simulink model "MCU_FOC"  (R2022b)
settings: Solver=FixedStepDiscrete  StartTime=0.0  StopTime=10.0  FixedStep=0.0001  RelTol=1e-3
values from neighbouring files (symbols this model uses):
  C_FOC_DecoupleEn_u8 = 0.0    [MCU_FOC_Sldd.sldd]    (also in MCU_FOC_Sldd_objects.m = myPackage.Parameter)
  C_FOC_DecoupleUdCoeff_f32 = 0.0    [MCU_FOC_Sldd.sldd]    (also in MCU_FOC_Sldd_objects.m = myPackage.Parameter)
  C_FOC_DecoupleUeCoeff_f32 = 0.0    [MCU_FOC_Sldd.sldd]    (also in MCU_FOC_Sldd_objects.m = myPackage.Parameter)
  C_FOC_DecoupleUqCoeff_f32 = 0.0    [MCU_FOC_Sldd.sldd]    (also in MCU_FOC_Sldd_objects.m = myPackage.Parameter)
  C_FOC_DPWMEN_u8 = 0.0    [MCU_FOC_Sldd.sldd]    (also in MCU_FOC_Sldd_objects.m = myPackage.Parameter)
  C_FOC_IgnoreShunt_u8 = 0.0    [MCU_FOC_Sldd.sldd]    (also in MCU_FOC_Sldd_objects.m = myPackage.Parameter)
  C_FOC_ThetaOffsetCoeff_f32 = 0.0    [MCU_FOC_Sldd.sldd]    (also in MCU_FOC_Sldd_objects.m = myPackage.Parameter)
undefined symbols (not defined in the file or in its folder): ABC_SAMPLE, ANALOG, cAgeingMode, cParaRecogMode, cSingleBoardMode, cVvvfOpenMode, MAIN_CPU_FRE, ParamCfg_BaseSpeed_u16, ParamCfg_CommandSource_u16, ParamCfg_IdKi_u16, ParamCfg_IdKp_u16, ParamCfg_IdStep1_u16, ParamCfg_IdStep2_u16, ParamCfg_IqKi_u16, ParamCfg_IqKp_u16, ParamCfg_IqStep_u16, ParamCfg_MotorLsd_u16, ParamCfg_MotorNp_u16, ParamCfg_MotorUlsq_u16, ParamCfg_PwmFreqHigh_u16, ParamCfg_PwmFreqLow_u16, ParamCfg_Pwmprdchgen_u16, ParamCfg_RotateNp_u16, ParamCfg_RotorFlux_u16, ParamCfg_SampleMode_u16, TESTBED
libraries: simulink x40, YS_UserDefined_Library x17
(part 2 of 2)

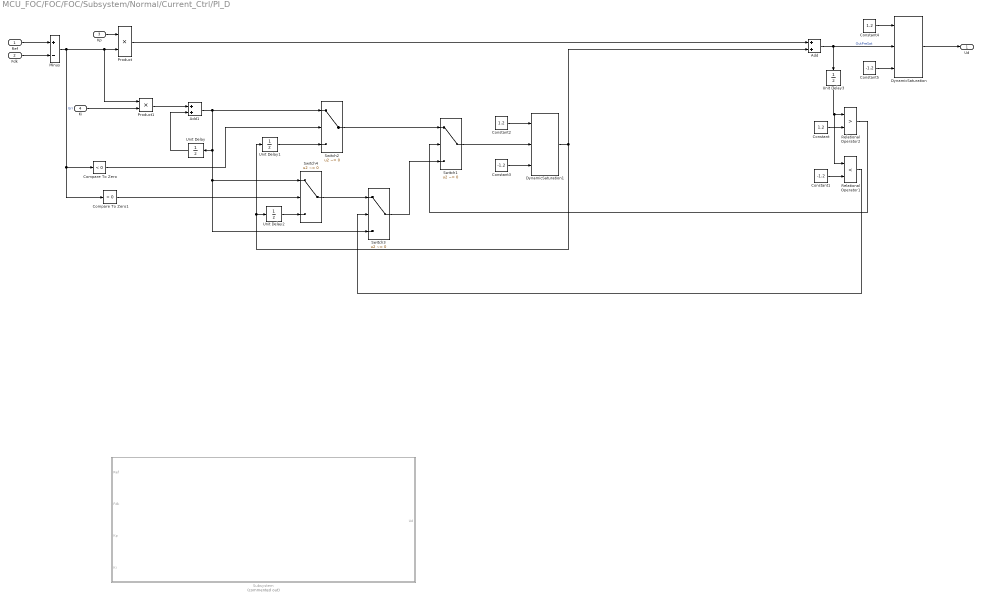
== system MCU_FOC/FOC/FOC/Subsystem/Normal/Current_Ctrl/PI_D ==
  Ref : Inport
  Fdk : Inport  Port=2
  Kp : Inport  Port=3
  Ki : Inport  Port=4
  Add : Sum
  Add1 : Sum
  Compare To Zero : simulink/Logic and Bit Operations/Compare To Zero  relop=<  OutDataTypeStr=boolean
  Compare To Zero1 : simulink/Logic and Bit Operations/Compare To Zero  relop=>  OutDataTypeStr=boolean
  Constant : Constant  Value=1.2  OutDataTypeStr=single
  Constant1 : Constant  Value=-1.2  OutDataTypeStr=single
  Constant2 : Constant  Value=1.2  OutDataTypeStr=single
  Constant3 : Constant  Value=-1.2  OutDataTypeStr=single
  Constant4 : Constant  Value=1.2  OutDataTypeStr=single
  Constant5 : Constant  Value=-1.2  OutDataTypeStr=single
  DynamicSaturation : YS_UserDefined_Library/Saturation/DynamicSaturation
      settings: SourceProductName=YS
  DynamicSaturation1 : YS_UserDefined_Library/Saturation/DynamicSaturation
      settings: SourceProductName=YS
  Minus : Sum  Inputs=+-
  Product : Product
  Product1 : Product
  Relational Operator1 : RelationalOperator  Operator=<  OutDataTypeStr=boolean  RndMeth=Simplest  InputSameDT=off
  Relational Operator2 : RelationalOperator  Operator=>  OutDataTypeStr=boolean  RndMeth=Simplest  InputSameDT=off
  Subsystem : Subsystem  Commented=on
  Switch{1..4} (4 alike) : Switch  Criteria=u2 ~= 0  SaturateOnIntegerOverflow=off  InputSameDT=off
  Unit Delay{,1..3} (4 alike) : UnitDelay  SampleTime=-1  HasFrameUpgradeWarning=on
  Ud : Outport
  wires:
  Constant2/1 -> DynamicSaturation1/1
  Constant/1 -> Relational Operator2/2
  Product/1 -> Add/1
  Ki/1 -> Product1/2
  Compare To Zero/1 -> Switch2/2
  DynamicSaturation1/1 -> Unit Delay1/1, Unit Delay2/1, Add/2
  Switch4/1 -> Switch3/1
  Unit Delay/1 -> Add1/2
  Switch2/1 -> Switch1/1
  Switch3/1 -> Switch1/3
  Compare To Zero1/1 -> Switch4/2
  Relational Operator1/1 -> Switch3/2
  Constant3/1 -> DynamicSaturation1/3
  Switch1/1 -> DynamicSaturation1/2
  Add1/1 -> Switch3/3, Switch4/1, Unit Delay/1, Switch2/1
  Unit Delay1/1 -> Switch2/3
  Add/1 -> DynamicSaturation/2, Unit Delay3/1  "OutPreSat"
  DynamicSaturation/1 -> Ud/1
  Product1/1 -> Add1/1
  Unit Delay2/1 -> Switch4/3
  Constant1/1 -> Relational Operator1/2
  Kp/1 -> Product/1
  Ref/1 -> Minus/1
  Minus/1 -> Product1/1, Product/2, Compare To Zero1/1, Compare To Zero/1  "Err"
  Fdk/1 -> Minus/2
  Constant4/1 -> DynamicSaturation/1
  Constant5/1 -> DynamicSaturation/3
  Relational Operator2/1 -> Switch1/2
  Unit Delay3/1 -> Relational Operator2/1, Relational Operator1/1

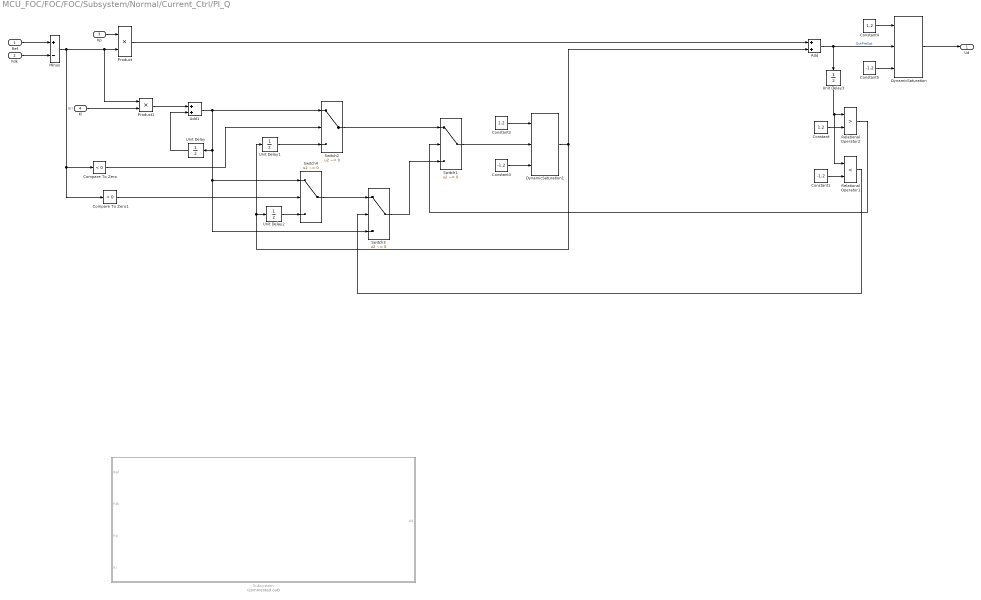
== system MCU_FOC/FOC/FOC/Subsystem/Normal/Current_Ctrl/PI_Q ==
  Ref : Inport
  Fdk : Inport  Port=2
  Kp : Inport  Port=3
  Ki : Inport  Port=4
  Add : Sum
  Add1 : Sum
  Compare To Zero : simulink/Logic and Bit Operations/Compare To Zero  relop=<  OutDataTypeStr=boolean
  Compare To Zero1 : simulink/Logic and Bit Operations/Compare To Zero  relop=>  OutDataTypeStr=boolean
  Constant : Constant  Value=1.2  OutDataTypeStr=single
  Constant1 : Constant  Value=-1.2  OutDataTypeStr=single
  Constant2 : Constant  Value=1.2  OutDataTypeStr=single
  Constant3 : Constant  Value=-1.2  OutDataTypeStr=single
  Constant4 : Constant  Value=1.2  OutDataTypeStr=single
  Constant5 : Constant  Value=-1.2  OutDataTypeStr=single
  DynamicSaturation : YS_UserDefined_Library/Saturation/DynamicSaturation
      settings: SourceProductName=YS
  DynamicSaturation1 : YS_UserDefined_Library/Saturation/DynamicSaturation
      settings: SourceProductName=YS
  Minus : Sum  Inputs=+-
  Product : Product
  Product1 : Product
  Relational Operator1 : RelationalOperator  Operator=<  OutDataTypeStr=boolean  RndMeth=Simplest  InputSameDT=off
  Relational Operator2 : RelationalOperator  Operator=>  OutDataTypeStr=boolean  RndMeth=Simplest  InputSameDT=off
  Subsystem : Subsystem  Commented=on
  Switch{1..4} (4 alike) : Switch  Criteria=u2 ~= 0  SaturateOnIntegerOverflow=off  InputSameDT=off
  Unit Delay{,1..3} (4 alike) : UnitDelay  SampleTime=-1  HasFrameUpgradeWarning=on
  Ud : Outport
  wires:
  Unit Delay3/1 -> Relational Operator1/1, Relational Operator2/1
  Relational Operator2/1 -> Switch1/2
  Constant5/1 -> DynamicSaturation/3
  Constant4/1 -> DynamicSaturation/1
  Fdk/1 -> Minus/2
  Minus/1 -> Compare To Zero/1, Compare To Zero1/1, Product/2, Product1/1  "Err"
  Ref/1 -> Minus/1
  Kp/1 -> Product/1
  Constant1/1 -> Relational Operator1/2
  Unit Delay2/1 -> Switch4/3
  Product1/1 -> Add1/1
  DynamicSaturation/1 -> Ud/1
  Add/1 -> Unit Delay3/1, DynamicSaturation/2  "OutPreSat"
  Unit Delay1/1 -> Switch2/3
  Add1/1 -> Switch2/1, Unit Delay/1, Switch4/1, Switch3/3
  Switch1/1 -> DynamicSaturation1/2
  Constant3/1 -> DynamicSaturation1/3
  Relational Operator1/1 -> Switch3/2
  Compare To Zero1/1 -> Switch4/2
  Switch3/1 -> Switch1/3
  Switch2/1 -> Switch1/1
  Unit Delay/1 -> Add1/2
  Switch4/1 -> Switch3/1
  DynamicSaturation1/1 -> Add/2, Unit Delay2/1, Unit Delay1/1
  Compare To Zero/1 -> Switch2/2
  Ki/1 -> Product1/2
  Product/1 -> Add/1
  Constant/1 -> Relational Operator2/2
  Constant2/1 -> DynamicSaturation1/1

== system MCU_FOC/FOC/FOC/Subsystem/Normal/Current_Ctrl/Step ==
  WorkCmdSourceModeCmd : Inport
  PwmPrdChg_PwmPrdCoffe : Inport  Port=2
  AgeingStep : Subsystem
  Compare To Constant1 : simulink/Logic and Bit Operations/Compare To Constant  relop===  const=cAgeingMode  OutDataTypeStr=boolean
  Logical Operator : Logic  Operator=NOT  AllPortsSameDT=off  OutDataTypeStr=boolean
  Merge : Merge
  Merge1 : Merge
  Merge2 : Merge
  Subsystem : Subsystem
  IdStep1 : Outport
  IdStep2 : Outport  Port=2
  IqStep : Outport  Port=3
  wires:
  WorkCmdSourceModeCmd/1 -> Compare To Constant1/1
  Compare To Constant1/1 -> Logical Operator/1, AgeingStep/Enable
  Logical Operator/1 -> Subsystem/Enable
  PwmPrdChg_PwmPrdCoffe/1 -> Subsystem/1(PwmPrdChg_PwmPrdCoffe)
  AgeingStep/1(IdStep1) -> Merge/1
  Subsystem/1(IdStep1) -> Merge/2
  AgeingStep/2(IdStep2) -> Merge1/1
  AgeingStep/3(IqStep) -> Merge2/1
  Subsystem/2(IdStep2) -> Merge1/2
  Subsystem/3(IqStep) -> Merge2/2
  Merge2/1 -> IqStep/1
  Merge1/1 -> IdStep2/1
  Merge/1 -> IdStep1/1

== system MCU_FOC/FOC/FOC/Subsystem/Normal/Current_Ctrl/TestBed ==
  Enable : EnablePort
  Constant : Constant  Value=ParamCfg_IdKp_u16  OutDataTypeStr=uint16
  Constant1 : Constant  Value=ParamCfg_IdKi_u16  OutDataTypeStr=uint16
  Constant2 : Constant  Value=ParamCfg_IqKp_u16  OutDataTypeStr=uint16
  Constant3 : Constant  Value=ParamCfg_IqKi_u16  OutDataTypeStr=uint16
  Data Type Conversion{,1..3} (4 alike) : DataTypeConversion  OutDataTypeStr=single  SaturateOnIntegerOverflow=off  RndMeth=Floor
  IdKpTestBed : Outport
  IdKiTestBed : Outport  Port=2
  IqKpTestBed : Outport  Port=3
  IqKiTestBed : Outport  Port=4
  wires:
  Constant3/1 -> Data Type Conversion3/1
  Constant/1 -> Data Type Conversion/1
  Constant1/1 -> Data Type Conversion1/1
  Constant2/1 -> Data Type Conversion2/1
  Data Type Conversion/1 -> IdKpTestBed/1
  Data Type Conversion1/1 -> IdKiTestBed/1
  Data Type Conversion2/1 -> IqKpTestBed/1
  Data Type Conversion3/1 -> IqKiTestBed/1

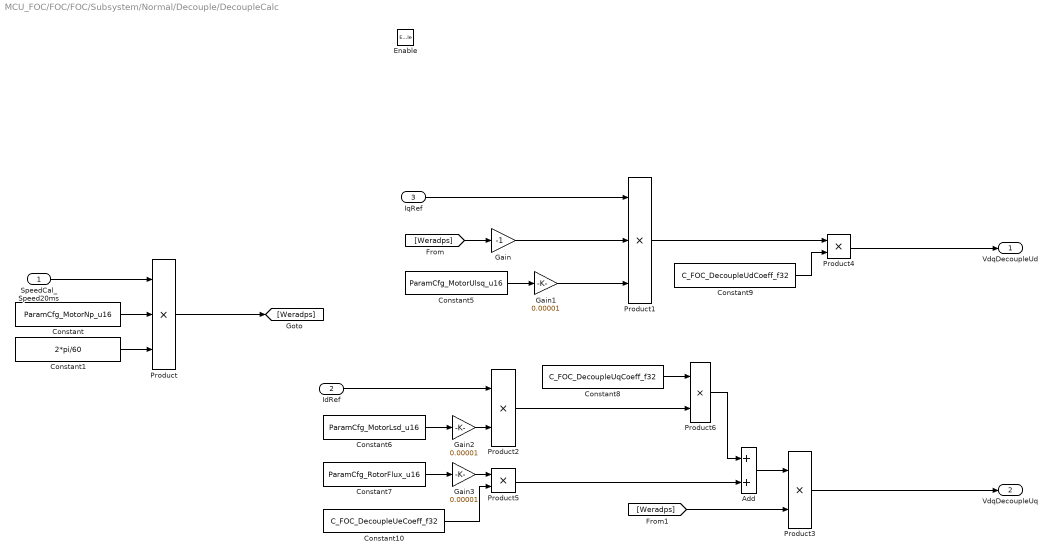
== system MCU_FOC/FOC/FOC/Subsystem/Normal/Decouple/DecoupleCalc ==
  SpeedCal_Speed20ms : Inport
  IdRef : Inport  Port=2
  IqRef : Inport  Port=3
  Enable : EnablePort
  Add : Sum  OutDataTypeStr=single
  Constant : Constant  Value=ParamCfg_MotorNp_u16  OutDataTypeStr=uint16
  Constant1 : Constant  Value=2*pi/60  OutDataTypeStr=single
      settings: AttributesFormatString=%<Description>0.1047197533
  Constant10 : Constant  Value=C_FOC_DecoupleUeCoeff_f32
  Constant5 : Constant  Value=ParamCfg_MotorUlsq_u16  OutDataTypeStr=uint16
  Constant6 : Constant  Value=ParamCfg_MotorLsd_u16  OutDataTypeStr=uint16
  Constant7 : Constant  Value=ParamCfg_RotorFlux_u16  OutDataTypeStr=uint16
  Constant8 : Constant  Value=C_FOC_DecoupleUqCoeff_f32
  Constant9 : Constant  Value=C_FOC_DecoupleUdCoeff_f32
  Gain : Gain  Gain=-1  ParamDataTypeStr=single  OutDataTypeStr=single
  Gain1 : Gain  Gain=0.00001  ParamDataTypeStr=single  OutDataTypeStr=single
  Gain2 : Gain  Gain=0.00001  ParamDataTypeStr=single  OutDataTypeStr=single
  Gain3 : Gain  Gain=0.00001  ParamDataTypeStr=single  OutDataTypeStr=single
  Product : Product  Inputs=3  OutDataTypeStr=single
  Product1 : Product  Inputs=3
  Product2 : Product  OutDataTypeStr=single
  Product{3..6} (4 alike) : Product
  VdqDecoupleUd : Outport  OutputWhenDisabled=reset  InitialOutput=0
  VdqDecoupleUq : Outport  Port=2  OutputWhenDisabled=reset  InitialOutput=0
  wires:
  Constant10/1 -> Product5/2
  Product6/1 -> Add/1
  Gain/1 -> Product1/2
  Product1/1 -> Product4/1
  Product4/1 -> VdqDecoupleUd/1
  Constant6/1 -> Gain2/1
  Gain3/1 -> Product5/1
  Constant9/1 -> Product4/2
  [Weradps] -> Gain/1
  IqRef/1 -> Product1/1
  Product3/1 -> VdqDecoupleUq/1
  Gain1/1 -> Product1/3
  Product2/1 -> Product6/2
  Constant7/1 -> Gain3/1
  Gain2/1 -> Product2/2
  Constant5/1 -> Gain1/1
  IdRef/1 -> Product2/1
  Product/1 -> [Weradps]
  SpeedCal_Speed20ms/1 -> Product/1
  Add/1 -> Product3/1
  Constant1/1 -> Product/3
  [Weradps] -> Product3/2
  Constant/1 -> Product/2
  Product5/1 -> Add/2
  Constant8/1 -> Product6/1

== system MCU_FOC/FOC/FOC/Subsystem/Normal/IdqGiveCal/AgeingMode ==
  WorkCmdCoreCurrentCmd : Inport
  WorkCmdTaskFreqCmd : Inport  Port=2
  WorkCmdCoreIdCmd : Inport  Port=3
  WorkCmdCoreIqCmd : Inport  Port=4
  Enable : EnablePort
  Chart : Stateflow chart  TreatAsAtomicUnit=on
  IdGiveAgeing : Outport
  IqAgeing : Outport  Port=2
  FreqAgeing : Outport  Port=3
  wires:
  WorkCmdCoreCurrentCmd/1 -> Chart/1(WorkCmdCoreCurrentCmd)
  WorkCmdCoreIdCmd/1 -> Chart/3(WorkCmdCoreIdCmd)
  WorkCmdCoreIqCmd/1 -> Chart/4(WorkCmdCoreIqCmd)
  WorkCmdTaskFreqCmd/1 -> Chart/2(WorkCmdTaskFreqCmd)
  Chart/1(Id) -> IdGiveAgeing/1
  Chart/2(Iq) -> IqAgeing/1
  Chart/3(AgentFreq) -> FreqAgeing/1

== system MCU_FOC/FOC/FOC/Subsystem/Normal/IdqGiveCal/ParaRecogMode ==
  ETheta_CurOut : Inport
  Enable : EnablePort
  Constant : Constant  Value=0  OutDataTypeStr=single
  IdGiveParaRecog : Outport
  IqGiveParaRecog : Outport  Port=2
  wires:
  ETheta_CurOut/1 -> IdGiveParaRecog/1
  Constant/1 -> IqGiveParaRecog/1

== system MCU_FOC/FOC/FOC/Subsystem/Normal/IdqGiveCal/VvvfMode ==
  ETheta_CurOut : Inport
  Enable : EnablePort
  Constant : Constant  Value=0  OutDataTypeStr=single
  IdGiveParaRecog : Outport
  IqGiveParaRecog : Outport  Port=2
  wires:
  Constant/1 -> IqGiveParaRecog/1
  ETheta_CurOut/1 -> IdGiveParaRecog/1

== system MCU_FOC/FOC/FOC/Subsystem/Normal/SVPWM/Enabled Subsystem ==
  Uaplha : Inport
  Ubeta : Inport  Port=2
  Enable : EnablePort
  1.732 : Gain  Gain=sqrt(3)
  sqrt(3) : Gain  Gain=sqrt(3)
  UalphaVvvvf : Outport
  UbetaVvvvf : Outport  Port=2
  wires:
  Uaplha/1 -> 1.732/1
  1.732/1 -> UalphaVvvvf/1
  Ubeta/1 -> sqrt(3)/1
  sqrt(3)/1 -> UbetaVvvvf/1

== system MCU_FOC/FOC/FOC/Subsystem/Normal/SVPWM/Enabled Subsystem1 ==
  Uaplha : Inport
  Ubeta : Inport  Port=2
  Enable : EnablePort
  UalphaNormal : Outport
  UbetaNormal : Outport  Port=2
  wires:
  Uaplha/1 -> UalphaNormal/1
  Ubeta/1 -> UbetaNormal/1

== system MCU_FOC/FOC/FOC/Subsystem/Normal/SVPWM/Subsystem ==
  UalphaSVPWM : Inport
  UbetaSVPWM : Inport  Port=2
  PwmPedChg_PwmPedReg : Inport  Port=3
  PwmPedChg_PwmPedRegH : Inport  Port=4
  Speed20msABS : Inport  Port=5
  Compare To Constant : simulink/Logic and Bit Operations/Compare To Constant  relop===  const=0  OutDataTypeStr=boolean
  Compare To Constant1 : simulink/Logic and Bit Operations/Compare To Constant  relop===  const=1  OutDataTypeStr=boolean
  DPWM : Subsystem
  DPWMEnJudge : Subsystem
  Merge : Merge
  Merge1 : Merge
  Merge2 : Merge
  SVPWMCal : Subsystem
  SVPWMCtrl : Subsystem
  Ta : Outport
  Tb : Outport  Port=2
  Tc : Outport  Port=3
  wires:
  UalphaSVPWM/1 -> DPWM/2(Ualpha), SVPWMCal/1(UalphaSVPWM)
  UbetaSVPWM/1 -> DPWM/3(Ubeta), SVPWMCal/2(UbetaSVPWM)
  PwmPedChg_PwmPedReg/1 -> SVPWMCtrl/4(PwmPedChg_PwmPedReg), DPWM/1(PwmPedReg)
  PwmPedChg_PwmPedRegH/1 -> SVPWMCtrl/5(PwmPedChg_PwmPedRegH)
  SVPWMCtrl/1(A) -> Ta/1
  SVPWMCtrl/2(B) -> Tb/1
  SVPWMCtrl/3(C) -> Tc/1
  Speed20msABS/1 -> DPWMEnJudge/1(Speed20msABS)
  Compare To Constant/1 -> SVPWMCal/Enable
  DPWMEnJudge/1(DPWMFlag) -> Compare To Constant1/1, Compare To Constant/1
  Compare To Constant1/1 -> DPWM/Enable
  SVPWMCal/1(Ta) -> Merge/1
  SVPWMCal/2(Tb) -> Merge2/1
  SVPWMCal/3(Tc) -> Merge1/1
  DPWM/1(Ta) -> Merge/2
  DPWM/2(Tb) -> Merge2/2
  DPWM/3(Tc) -> Merge1/2
  Merge/1 -> SVPWMCtrl/1(Ta)
  Merge2/1 -> SVPWMCtrl/2(Tb)
  Merge1/1 -> SVPWMCtrl/3(Tc)

== system MCU_FOC/FOC/FOC/Subsystem/Normal/CurrentCal/Enabled Subsystem/CurrentRegen ==
  IgnoreShunt : Inport
  Ia : Inport  Port=2
  Ib : Inport  Port=3
  Ic : Inport  Port=4
  AB : Subsystem  TreatAsAtomicUnit=on
  AC : Subsystem  TreatAsAtomicUnit=on
  BC : Subsystem  TreatAsAtomicUnit=on
  IgnoreA : simulink/Logic and Bit Operations/Compare To Constant  relop===  const=1  OutDataTypeStr=boolean
  IgnoreB : simulink/Logic and Bit Operations/Compare To Constant  relop===  const=2  OutDataTypeStr=boolean
  IgnoreC : simulink/Logic and Bit Operations/Compare To Constant  relop===  const=3  OutDataTypeStr=boolean
  Merge : Merge  Inputs=3
  Merge1 : Merge  Inputs=3
  Merge2 : Merge  Inputs=3
  IaRegen : Outport
  IbRegen : Outport  Port=2
  IcRegen : Outport  Port=3
  wires:
  IgnoreShunt/1 -> IgnoreC/1, IgnoreB/1, IgnoreA/1
  Ia/1 -> AB/1(Ia), AC/1(Ia), BC/1(Ia)
  Ib/1 -> AB/2(Ib), AC/2(Ib), BC/2(Ib)
  Ic/1 -> AB/3(Ic), AC/3(Ic), BC/3(Ic)
  IgnoreA/1 -> BC/Enable
  IgnoreB/1 -> AC/Enable
  IgnoreC/1 -> AB/Enable
  BC/1(IaRegen) -> Merge/1
  AC/1(IaRegen) -> Merge/2
  AB/1(IaRegen) -> Merge/3
  BC/2(IbRegen) -> Merge1/1
  AC/2(IbRegen) -> Merge1/2
  AB/2(IbRegen) -> Merge1/3
  AB/3(IcRegen) -> Merge2/3
  AC/3(IcRegen) -> Merge2/2
  BC/3(IcRegen) -> Merge2/1
  Merge/1 -> IaRegen/1
  Merge1/1 -> IbRegen/1
  Merge2/1 -> IcRegen/1

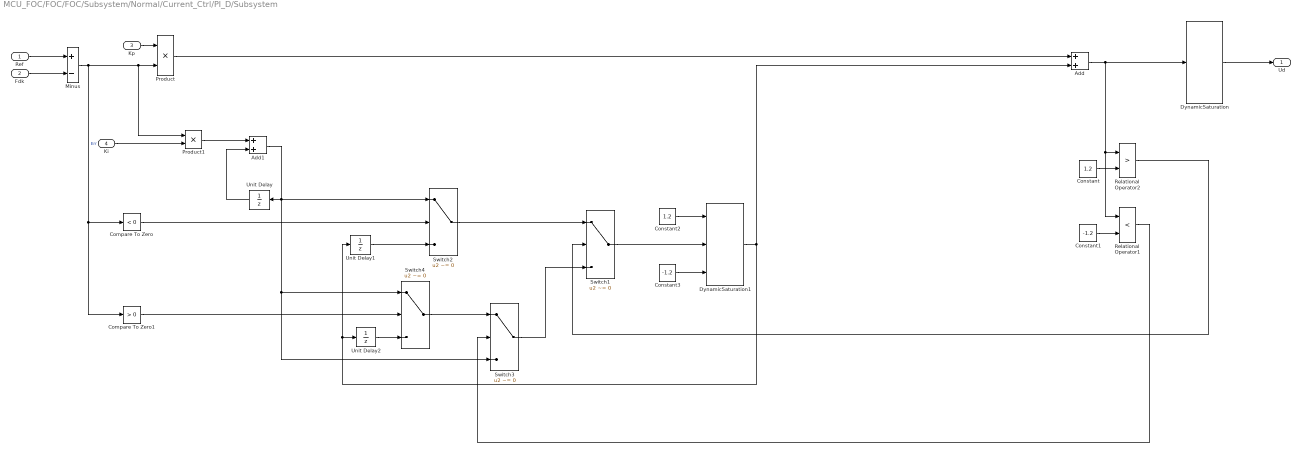
== system MCU_FOC/FOC/FOC/Subsystem/Normal/Current_Ctrl/PI_D/Subsystem ==
  Ref : Inport
  Fdk : Inport  Port=2
  Kp : Inport  Port=3
  Ki : Inport  Port=4
  Add : Sum
  Add1 : Sum
  Compare To Zero : simulink/Logic and Bit Operations/Compare To Zero  relop=<  OutDataTypeStr=boolean
  Compare To Zero1 : simulink/Logic and Bit Operations/Compare To Zero  relop=>  OutDataTypeStr=boolean
  Constant : Constant  Value=1.2  OutDataTypeStr=single
  Constant1 : Constant  Value=-1.2  OutDataTypeStr=single
  Constant2 : Constant  Value=1.2  OutDataTypeStr=single
  Constant3 : Constant  Value=-1.2  OutDataTypeStr=single
  DynamicSaturation : YS_UserDefined_Library/Saturation/DynamicSaturation
      settings: SourceProductName=YS
  DynamicSaturation1 : YS_UserDefined_Library/Saturation/DynamicSaturation
      settings: SourceProductName=YS
  Minus : Sum  Inputs=+-
  Product : Product
  Product1 : Product
  Relational Operator1 : RelationalOperator  Operator=<  OutDataTypeStr=boolean  RndMeth=Simplest  InputSameDT=off
  Relational Operator2 : RelationalOperator  Operator=>  OutDataTypeStr=boolean  RndMeth=Simplest  InputSameDT=off
  Switch{1..4} (4 alike) : Switch  Criteria=u2 ~= 0  SaturateOnIntegerOverflow=off  InputSameDT=off
  Unit Delay : UnitDelay  SampleTime=-1  HasFrameUpgradeWarning=on
  Unit Delay1 : UnitDelay  SampleTime=-1  HasFrameUpgradeWarning=on
  Unit Delay2 : UnitDelay  SampleTime=-1  HasFrameUpgradeWarning=on
  Ud : Outport
  wires:
  Unit Delay/1 -> Add1/2
  Ki/1 -> Product1/2
  Product/1 -> Add/1
  Constant/1 -> Relational Operator2/2
  Kp/1 -> Product/1
  Minus/1 -> Product1/1, Product/2, Compare To Zero1/1, Compare To Zero/1  "Err"
  Add/1 -> Relational Operator2/1, Relational Operator1/1, DynamicSaturation/2
  DynamicSaturation/1 -> Ud/1
  Fdk/1 -> Minus/2
  Constant1/1 -> Relational Operator1/2
  Ref/1 -> Minus/1
  Product1/1 -> Add1/1
  Add1/1 -> Switch3/3, Switch4/1, Switch2/1, Unit Delay/1
  Relational Operator2/1 -> Switch1/2
  Switch2/1 -> Switch1/1
  Compare To Zero/1 -> Switch2/2
  Unit Delay1/1 -> Switch2/3
  Switch3/1 -> Switch1/3
  Relational Operator1/1 -> Switch3/2
  Switch4/1 -> Switch3/1
  Compare To Zero1/1 -> Switch4/2
  Unit Delay2/1 -> Switch4/3
  Switch1/1 -> DynamicSaturation1/2
  Constant2/1 -> DynamicSaturation1/1
  Constant3/1 -> DynamicSaturation1/3
  DynamicSaturation1/1 -> Unit Delay1/1, Unit Delay2/1, Add/2

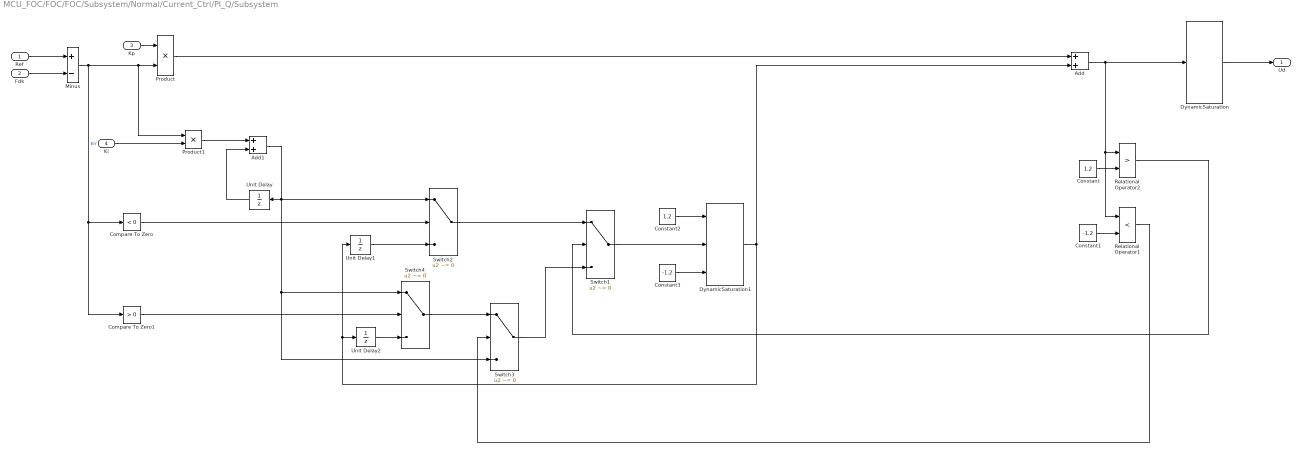
== system MCU_FOC/FOC/FOC/Subsystem/Normal/Current_Ctrl/PI_Q/Subsystem ==
  Ref : Inport
  Fdk : Inport  Port=2
  Kp : Inport  Port=3
  Ki : Inport  Port=4
  Add : Sum
  Add1 : Sum
  Compare To Zero : simulink/Logic and Bit Operations/Compare To Zero  relop=<  OutDataTypeStr=boolean
  Compare To Zero1 : simulink/Logic and Bit Operations/Compare To Zero  relop=>  OutDataTypeStr=boolean
  Constant : Constant  Value=1.2  OutDataTypeStr=single
  Constant1 : Constant  Value=-1.2  OutDataTypeStr=single
  Constant2 : Constant  Value=1.2  OutDataTypeStr=single
  Constant3 : Constant  Value=-1.2  OutDataTypeStr=single
  DynamicSaturation : YS_UserDefined_Library/Saturation/DynamicSaturation
      settings: SourceProductName=YS
  DynamicSaturation1 : YS_UserDefined_Library/Saturation/DynamicSaturation
      settings: SourceProductName=YS
  Minus : Sum  Inputs=+-
  Product : Product
  Product1 : Product
  Relational Operator1 : RelationalOperator  Operator=<  OutDataTypeStr=boolean  RndMeth=Simplest  InputSameDT=off
  Relational Operator2 : RelationalOperator  Operator=>  OutDataTypeStr=boolean  RndMeth=Simplest  InputSameDT=off
  Switch{1..4} (4 alike) : Switch  Criteria=u2 ~= 0  SaturateOnIntegerOverflow=off  InputSameDT=off
  Unit Delay : UnitDelay  SampleTime=-1  HasFrameUpgradeWarning=on
  Unit Delay1 : UnitDelay  SampleTime=-1  HasFrameUpgradeWarning=on
  Unit Delay2 : UnitDelay  SampleTime=-1  HasFrameUpgradeWarning=on
  Ud : Outport
  wires:
  DynamicSaturation1/1 -> Add/2, Unit Delay2/1, Unit Delay1/1
  Constant3/1 -> DynamicSaturation1/3
  Constant2/1 -> DynamicSaturation1/1
  Switch1/1 -> DynamicSaturation1/2
  Unit Delay2/1 -> Switch4/3
  Compare To Zero1/1 -> Switch4/2
  Switch4/1 -> Switch3/1
  Relational Operator1/1 -> Switch3/2
  Switch3/1 -> Switch1/3
  Unit Delay1/1 -> Switch2/3
  Compare To Zero/1 -> Switch2/2
  Switch2/1 -> Switch1/1
  Relational Operator2/1 -> Switch1/2
  Add1/1 -> Unit Delay/1, Switch2/1, Switch4/1, Switch3/3
  Product1/1 -> Add1/1
  Ref/1 -> Minus/1
  Constant1/1 -> Relational Operator1/2
  Fdk/1 -> Minus/2
  DynamicSaturation/1 -> Ud/1
  Add/1 -> DynamicSaturation/2, Relational Operator1/1, Relational Operator2/1
  Minus/1 -> Compare To Zero/1, Compare To Zero1/1, Product/2, Product1/1  "Err"
  Kp/1 -> Product/1
  Constant/1 -> Relational Operator2/2
  Product/1 -> Add/1
  Ki/1 -> Product1/2
  Unit Delay/1 -> Add1/2

== system MCU_FOC/FOC/FOC/Subsystem/Normal/Current_Ctrl/Step/AgeingStep ==
  Enable : EnablePort
  Constant : Constant  Value=0.02  OutDataTypeStr=single
  IdStep1 : Outport
  IdStep2 : Outport  Port=2
  IqStep : Outport  Port=3
  wires:
  Constant/1 -> IqStep/1, IdStep2/1, IdStep1/1

== system MCU_FOC/FOC/FOC/Subsystem/Normal/Current_Ctrl/Step/Subsystem ==
  PwmPrdChg_PwmPrdCoffe : Inport
  Enable : EnablePort
  Compare To Constant : simulink/Logic and Bit Operations/Compare To Constant  relop===  const=TESTBED  OutDataTypeStr=boolean
  Constant : Constant  Value=ParamCfg_CommandSource_u16  OutDataTypeStr=uint16
  Constant1 : Constant  Value=0.0001  OutDataTypeStr=single
  Constant2 : Constant  Value=10  OutDataTypeStr=single
  Constant3 : Constant  Value=ParamCfg_IdStep1_u16  OutDataTypeStr=uint16
  Constant4 : Constant  Value=ParamCfg_IdStep2_u16  OutDataTypeStr=uint16
  Constant5 : Constant  Value=ParamCfg_IqStep_u16  OutDataTypeStr=uint16
  Product : Product  Inputs=3  OutDataTypeStr=single
  Product1 : Product  Inputs=3  OutDataTypeStr=single
  Product2 : Product  Inputs=3  OutDataTypeStr=single
  Switch : Switch  Criteria=u2 ~= 0  SaturateOnIntegerOverflow=off  InputSameDT=off
  Switch1 : Switch  Criteria=u2 ~= 0  SaturateOnIntegerOverflow=off  InputSameDT=off
  Switch2 : Switch  Criteria=u2 ~= 0  SaturateOnIntegerOverflow=off  InputSameDT=off
  IdStep1 : Outport
  IdStep2 : Outport  Port=2
  IqStep : Outport  Port=3
  wires:
  Constant/1 -> Compare To Constant/1
  Compare To Constant/1 -> Switch/2, Switch1/2, Switch2/2
  Switch/1 -> IdStep1/1
  Switch1/1 -> IdStep2/1
  Switch2/1 -> IqStep/1
  Constant2/1 -> Switch2/3, Switch1/3, Switch/3
  Constant3/1 -> Product/2
  Constant1/1 -> Product2/2, Product1/2, Product/3
  PwmPrdChg_PwmPrdCoffe/1 -> Product2/1, Product1/1, Product/1
  Product/1 -> Switch/1
  Constant4/1 -> Product1/3
  Product1/1 -> Switch1/1
  Product2/1 -> Switch2/1
  Constant5/1 -> Product2/3

== system MCU_FOC/FOC/FOC/Subsystem/Normal/IdqGiveCal/AgeingMode/Chart/Slope ==
  Ref : Inport  OutDataTypeStr=double  PortDimensions=1
  step : Inport  Port=2  OutDataTypeStr=double  PortDimensions=1
  f : TriggerPort  TriggerType=function-call  VariantControl=(inherit)
      settings: CopyFcn=Stateflow.SLINSF.SimulinkMan.removeBlockPreDeleteFcn  PreDeleteFcn=Stateflow.SLINSF.SimulinkMan.unsafePredeleteFcn
  Add : Sum
  Gain : Gain  Gain=-1  ParamDataTypeStr=single  OutDataTypeStr=single
  Minus : Sum  Inputs=+-
  Minus1 : Sum  Inputs=+-
  Relational Operator : RelationalOperator  Operator=>  OutDataTypeStr=boolean  RndMeth=Simplest  InputSameDT=off
  Relational Operator1 : RelationalOperator  Operator=<  OutDataTypeStr=boolean  RndMeth=Simplest  InputSameDT=off
  Switch : Switch  Criteria=u2 ~= 0  SaturateOnIntegerOverflow=off  InputSameDT=off
  Switch1 : Switch  Criteria=u2 ~= 0  SaturateOnIntegerOverflow=off  InputSameDT=off
  Unit Delay : UnitDelay  SampleTime=-1  HasFrameUpgradeWarning=on
  Act : Outport
  wires:
  Ref/1 -> Switch1/3, Minus/1
  Unit Delay/1 -> Add/1, Minus1/1, Minus/2
  Minus/1 -> Relational Operator1/1, Relational Operator/1
  step/1 -> Gain/1, Minus1/2, Add/2, Relational Operator/2
  Relational Operator/1 -> Switch/2
  Add/1 -> Switch/1
  Switch/1 -> Unit Delay/1, Act/1
  Gain/1 -> Relational Operator1/2
  Relational Operator1/1 -> Switch1/2
  Switch1/1 -> Switch/3
  Minus1/1 -> Switch1/1

== system MCU_FOC/FOC/FOC/Subsystem/Normal/SVPWM/Subsystem/DPWM ==
  PwmPedReg : Inport
  Ualpha : Inport  Port=2
  Ubeta : Inport  Port=3
  Enable : EnablePort
  Constant : Constant  Value=700  OutDataTypeStr=single
  Divide : Product  Inputs=*/  OutDataTypeStr=single
  MATLAB Function : MATLAB Function  TreatAsAtomicUnit=on
  Ta : Outport
  Tb : Outport  Port=2
  Tc : Outport  Port=3
  wires:
  Ualpha/1 -> MATLAB Function/2(Ualpha)
  Ubeta/1 -> MATLAB Function/3(Ubeta)
  Divide/1 -> MATLAB Function/1(TMin)
  MATLAB Function/1(Ta) -> Ta/1
  MATLAB Function/2(Tb) -> Tb/1
  MATLAB Function/3(Tc) -> Tc/1
  Constant/1 -> Divide/1
  PwmPedReg/1 -> Divide/2

== system MCU_FOC/FOC/FOC/Subsystem/Normal/SVPWM/Subsystem/DPWMEnJudge ==
  Speed20msABS : Inport
  Compare To Constant : simulink/Logic and Bit Operations/Compare To Constant  relop===  const=0  OutDataTypeStr=boolean
  Compare To Constant1 : simulink/Logic and Bit Operations/Compare To Constant  relop===  const=1  OutDataTypeStr=boolean
  Constant : Constant  Value=C_FOC_DPWMEN_u8  OutDataTypeStr=uint8
  Constant1 : Constant  Value=0  OutDataTypeStr=uint8
  Constant2 : Constant  Value=ParamCfg_BaseSpeed_u16  OutDataTypeStr=uint16
  Constant3 : Constant  OutDataTypeStr=uint8
  Constant4 : Constant  Value=0  OutDataTypeStr=uint8
  Logical Operator : Logic  AllPortsSameDT=off  OutDataTypeStr=boolean
  Logical Operator1 : Logic  AllPortsSameDT=off  OutDataTypeStr=boolean
  Relational Operator : RelationalOperator  OutDataTypeStr=boolean  RndMeth=Simplest  InputSameDT=off
  Relational Operator1 : RelationalOperator  Operator=<=  OutDataTypeStr=boolean  RndMeth=Simplest  InputSameDT=off
  Switch : Switch  Criteria=u2 ~= 0  SaturateOnIntegerOverflow=off  InputSameDT=off
  Switch1 : Switch  Criteria=u2 ~= 0  SaturateOnIntegerOverflow=off  InputSameDT=off
  Switch2 : Switch  Criteria=u2 ~= 0  SaturateOnIntegerOverflow=off  InputSameDT=off
  Unit Delay : UnitDelay  SampleTime=-1  HasFrameUpgradeWarning=on
  DPWMFlag : Outport
  wires:
  Constant/1 -> Switch/2
  Constant1/1 -> Switch/1
  Speed20msABS/1 -> Relational Operator1/1, Relational Operator/1
  Constant2/1 -> Relational Operator1/2, Relational Operator/2
  Switch/1 -> Unit Delay/1, DPWMFlag/1
  Relational Operator/1 -> Logical Operator/1
  Compare To Constant/1 -> Logical Operator/2
  Unit Delay/1 -> Switch2/3, Compare To Constant1/1, Compare To Constant/1
  Logical Operator/1 -> Switch1/2
  Switch1/1 -> Switch/3
  Constant3/1 -> Switch1/1
  Compare To Constant1/1 -> Logical Operator1/1
  Relational Operator1/1 -> Logical Operator1/2
  Logical Operator1/1 -> Switch2/2
  Constant4/1 -> Switch2/1

== system MCU_FOC/FOC/FOC/Subsystem/Normal/SVPWM/Subsystem/SVPWMCal ==
  UalphaSVPWM : Inport
  UbetaSVPWM : Inport  Port=2
  Enable : EnablePort
  ActionTimeCal : Subsystem
  N Caculate : Subsystem  Commented=on
  SectorJudgement : Subsystem
  SectorTransfer : Subsystem
  Subsystem : Subsystem
  SwitchTime : Subsystem
  Ta : Outport
  Tb : Outport  Port=2
  Tc : Outport  Port=3
  wires:
  UbetaSVPWM/1 -> SectorJudgement/2(Ubeta)
  ActionTimeCal/1(T1) -> Subsystem/1(T1)  "T1"
  SwitchTime/3(Tcm3) -> Tc/1
  SwitchTime/2(Tcm2) -> Tb/1
  SectorJudgement/1(OriginalSector) -> SectorTransfer/1(OriginalSector)
  SectorTransfer/1(realSector) -> SwitchTime/3(realSector), ActionTimeCal/1(realSector)  "sector"
  ActionTimeCal/2(T2) -> Subsystem/2(T2)  "T2"
  SectorJudgement/2(sqrt(3)/2Alpha) -> ActionTimeCal/2(sqrt(3)/2Alpha)
  UalphaSVPWM/1 -> SectorJudgement/1(Ualpha)
  SwitchTime/1(Tcm1) -> Ta/1
  SectorJudgement/3(-1/2Beta) -> ActionTimeCal/3(-1/2Beta)
  Subsystem/1(T1Final) -> SwitchTime/1(T1Final)
  Subsystem/2(T2Final) -> SwitchTime/2(T2Final)

== system MCU_FOC/FOC/FOC/Subsystem/Normal/SVPWM/Subsystem/SVPWMCtrl ==
  Ta : Inport
  Tb : Inport  Port=2
  Tc : Inport  Port=3
  PwmPedChg_PwmPedReg : Inport  Port=4
  PwmPedChg_PwmPedRegH : Inport  Port=5
  Data Type Conversion : DataTypeConversion  OutDataTypeStr=uint16  SaturateOnIntegerOverflow=off  RndMeth=Floor
  Data Type Conversion1 : DataTypeConversion  OutDataTypeStr=uint16  SaturateOnIntegerOverflow=off  RndMeth=Floor
  Data Type Conversion2 : DataTypeConversion  OutDataTypeStr=uint16  SaturateOnIntegerOverflow=off  RndMeth=Floor
  DynamicSaturation : YS_UserDefined_Library/Saturation/DynamicSaturation
      settings: SourceProductName=YS
  DynamicSaturation1 : YS_UserDefined_Library/Saturation/DynamicSaturation
      settings: SourceProductName=YS
  DynamicSaturation2 : YS_UserDefined_Library/Saturation/DynamicSaturation
      settings: SourceProductName=YS
  PWM_PERIOD_L : Constant  Value=700  OutDataTypeStr=uint16
  Product : Product
  Product1 : Product
  Product2 : Product
  A : Outport
  B : Outport  Port=2
  C : Outport  Port=3
  wires:
  Ta/1 -> Product/1
  Tc/1 -> Product2/1
  Tb/1 -> Product1/1
  PwmPedChg_PwmPedReg/1 -> Product/2, Product1/2, Product2/2
  Product/1 -> Data Type Conversion/1
  Product1/1 -> Data Type Conversion1/1
  Product2/1 -> Data Type Conversion2/1
  Data Type Conversion/1 -> DynamicSaturation/2
  PwmPedChg_PwmPedRegH/1 -> DynamicSaturation2/1, DynamicSaturation1/1, DynamicSaturation/1
  PWM_PERIOD_L/1 -> DynamicSaturation2/3, DynamicSaturation1/3, DynamicSaturation/3
  Data Type Conversion1/1 -> DynamicSaturation1/2
  Data Type Conversion2/1 -> DynamicSaturation2/2
  DynamicSaturation1/1 -> B/1
  DynamicSaturation/1 -> A/1
  DynamicSaturation2/1 -> C/1

== system MCU_FOC/FOC/FOC/Subsystem/Normal/CurrentCal/Enabled Subsystem/CurrentRegen/AB ==
  Ia : Inport
  Ib : Inport  Port=2
  Ic : Inport  Port=3
  Enable : EnablePort
  Add : Sum
  Data Type Duplicate : DataTypeDuplicate  NumInputPorts=3
  Gain : Gain  Gain=-1  OutDataTypeStr=single
  Gain1 : Gain  Gain=-1  OutDataTypeStr=single
  Terminator : Terminator
  IaRegen : Outport
  IbRegen : Outport  Port=2
  IcRegen : Outport  Port=3
  wires:
  Ia/1 -> Gain/1, Data Type Duplicate/1, IaRegen/1
  Ib/1 -> Gain1/1, Data Type Duplicate/2, IbRegen/1
  Ic/1 -> Terminator/1
  Gain/1 -> Add/1
  Gain1/1 -> Add/2
  Add/1 -> Data Type Duplicate/3, IcRegen/1

== system MCU_FOC/FOC/FOC/Subsystem/Normal/CurrentCal/Enabled Subsystem/CurrentRegen/AC ==
  Ia : Inport
  Ib : Inport  Port=2
  Ic : Inport  Port=3
  Enable : EnablePort
  Add : Sum
  Data Type Duplicate : DataTypeDuplicate  NumInputPorts=3
  Gain : Gain  Gain=-1  OutDataTypeStr=single
  Gain1 : Gain  Gain=-1  OutDataTypeStr=single
  Terminator : Terminator
  IaRegen : Outport
  IbRegen : Outport  Port=2
  IcRegen : Outport  Port=3
  wires:
  Ia/1 -> Gain/1, Data Type Duplicate/1, IaRegen/1
  Ib/1 -> Terminator/1
  Ic/1 -> Data Type Duplicate/3, IcRegen/1, Gain1/1
  Gain/1 -> Add/1
  Gain1/1 -> Add/2
  Add/1 -> Data Type Duplicate/2, IbRegen/1

== system MCU_FOC/FOC/FOC/Subsystem/Normal/CurrentCal/Enabled Subsystem/CurrentRegen/BC ==
  Ia : Inport
  Ib : Inport  Port=2
  Ic : Inport  Port=3
  Enable : EnablePort
  Add : Sum
  Data Type Duplicate : DataTypeDuplicate  NumInputPorts=3
  Gain : Gain  Gain=-1  OutDataTypeStr=single
  Gain1 : Gain  Gain=-1  OutDataTypeStr=single
  Terminator : Terminator
  IaRegen : Outport
  IbRegen : Outport  Port=2
  IcRegen : Outport  Port=3
  wires:
  Ia/1 -> Terminator/1
  Ib/1 -> Gain/1, Data Type Duplicate/2, IbRegen/1
  Ic/1 -> Gain1/1, Data Type Duplicate/3, IcRegen/1
  Gain/1 -> Add/1
  Gain1/1 -> Add/2
  Add/1 -> Data Type Duplicate/1, IaRegen/1

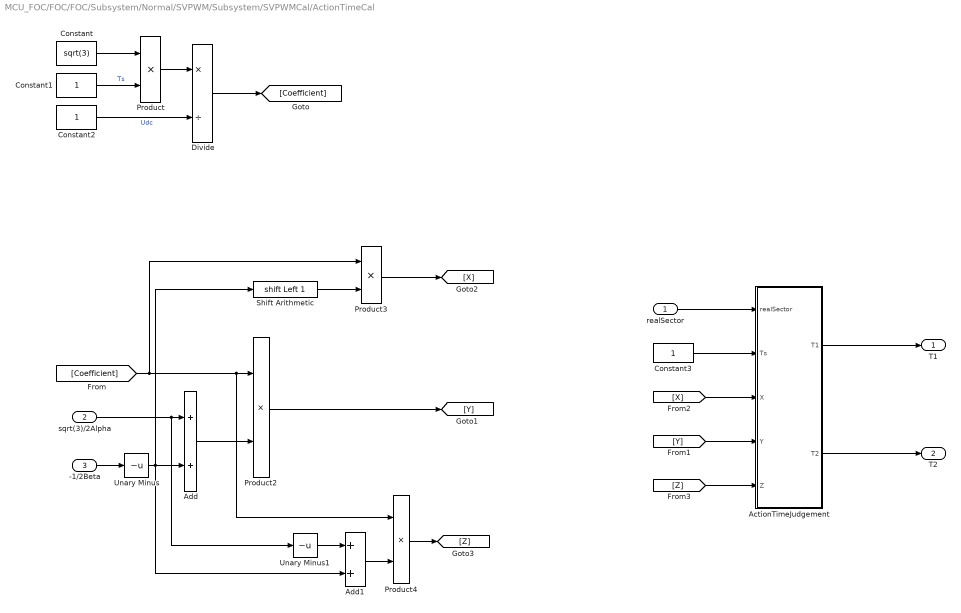
== system MCU_FOC/FOC/FOC/Subsystem/Normal/SVPWM/Subsystem/SVPWMCal/ActionTimeCal ==
  realSector : Inport
  sqrt(3)/2Alpha : Inport  Port=2
  -1/2Beta : Inport  Port=3
  ActionTimeJudgement : MATLAB Function  TreatAsAtomicUnit=on
  Add : Sum
  Add1 : Sum
  Constant : Constant  Value=sqrt(3)  OutDataTypeStr=single
  Constant1 : Constant  OutDataTypeStr=single
  Constant2 : Constant  OutDataTypeStr=single
  Constant3 : Constant  OutDataTypeStr=single
  Divide : Product  Inputs=*/
  Product{,2..4} (4 alike) : Product
  Shift Arithmetic : ArithShift  BitShiftNumber=1  BitShiftDirection=Left
  Unary Minus : UnaryMinus
  Unary Minus1 : UnaryMinus
  T1 : Outport
  T2 : Outport  Port=2
  wires:
  Constant/1 -> Product/1
  Constant1/1 -> Product/2  "Ts"
  Product/1 -> Divide/1
  Divide/1 -> [Coefficient]
  [Coefficient] -> Product3/1, Product4/1, Product2/1
  sqrt(3)/2Alpha/1 -> Unary Minus1/1, Add/1
  -1/2Beta/1 -> Unary Minus/1
  Unary Minus/1 -> Add1/2, Add/2, Shift Arithmetic/1
  Add/1 -> Product2/2
  Product2/1 -> [Y]
  Shift Arithmetic/1 -> Product3/2
  Product3/1 -> [X]
  Unary Minus1/1 -> Add1/1
  Add1/1 -> Product4/2
  Product4/1 -> [Z]
  [X] -> ActionTimeJudgement/3(X)
  [Y] -> ActionTimeJudgement/4(Y)
  [Z] -> ActionTimeJudgement/5(Z)
  realSector/1 -> ActionTimeJudgement/1(realSector)
  ActionTimeJudgement/1(T1) -> T1/1
  ActionTimeJudgement/2(T2) -> T2/1
  Constant3/1 -> ActionTimeJudgement/2(Ts)
  Constant2/1 -> Divide/2  "Udc"

== system MCU_FOC/FOC/FOC/Subsystem/Normal/SVPWM/Subsystem/SVPWMCal/N Caculate ==
  beta : Inport
  alpha : Inport  Port=2
  Add : Sum  Inputs=+-
  Add1 : Sum  Inputs=--
  Add2 : Sum  Inputs=+++
  Constant : Constant
  Constant1 : Constant  Value=0
  Gain : Gain  Gain=sqrt(3)/2
  Gain1 : Gain  Gain=1/2
  Gain2 : Gain  Gain=4
  Gain3 : Gain  Gain=2
  Gain4 : Gain
  MATLAB Function : MATLAB Function  TreatAsAtomicUnit=on
  Switch : Switch  Criteria=u2 > Threshold  SaturateOnIntegerOverflow=off  InputSameDT=off
  Switch1 : Switch  Criteria=u2 > Threshold  SaturateOnIntegerOverflow=off  InputSameDT=off
  Switch2 : Switch  Criteria=u2 > Threshold  SaturateOnIntegerOverflow=off  InputSameDT=off
  N : Outport  VectorParamsAs1DForOutWhenUnconnected=off
  wires:
  Switch/1 -> Gain4/1  "A"
  Add/1 -> Switch1/2
  Gain/1 -> Add1/1, Add/1
  Gain3/1 -> Add2/2
  Gain2/1 -> Add2/3
  Constant/1 -> Switch/1, Switch2/1, Switch1/1
  Add1/1 -> Switch2/2
  Gain1/1 -> Add1/2, Add/2
  Add2/1 -> MATLAB Function/1(u)
  Constant1/1 -> Switch2/3, Switch1/3, Switch/3
  Gain4/1 -> Add2/1
  beta/1 -> Switch/2, Gain1/1
  Switch2/1 -> Gain2/1  "C"
  Switch1/1 -> Gain3/1  "B"
  alpha/1 -> Gain/1
  MATLAB Function/1(y) -> N/1

== system MCU_FOC/FOC/FOC/Subsystem/Normal/SVPWM/Subsystem/SVPWMCal/SectorJudgement ==
  Ualpha : Inport
  Ubeta : Inport  Port=2
  Add : Sum
  Add1 : Sum
  Add2 : Sum  Inputs=3
  Compare To Zero : simulink/Logic and Bit Operations/Compare To Zero  relop=>  OutDataTypeStr=uint8
  Compare To Zero1 : simulink/Logic and Bit Operations/Compare To Zero  relop=>  OutDataTypeStr=uint8
  Compare To Zero2 : simulink/Logic and Bit Operations/Compare To Zero  relop=>  OutDataTypeStr=uint8
  Constant : Constant  Value=sqrt(3)/2  OutDataTypeStr=single
  Constant1 : Constant  Value=-1/2  OutDataTypeStr=single
  Constant2 : Constant  Value=-1  OutDataTypeStr=single
  Product : Product
  Product1 : Product
  Product2 : Product
  Shift Arithmetic : ArithShift  BitShiftNumber=2  BitShiftDirection=Left
  Shift Arithmetic1 : ArithShift  BitShiftNumber=1  BitShiftDirection=Left
  OriginalSector : Outport
  sqrt(3)/2Alpha : Outport  Port=2
  -1/2Beta : Outport  Port=3
  wires:
  Ubeta/1 -> Product1/2, [Vref1]
  Ualpha/1 -> Product/1
  Constant/1 -> Product/2
  Constant1/1 -> Product1/1
  Product/1 -> sqrt(3)/2Alpha/1, Product2/1, Add/1
  Product1/1 -> -1/2Beta/1, Add1/2, Add/2
  Add/1 -> [Vref2]
  Constant2/1 -> Product2/2
  Product2/1 -> Add1/1
  Add1/1 -> [Vref3]
  [Vref3] -> Compare To Zero2/1
  [Vref2] -> Compare To Zero1/1
  Shift Arithmetic1/1 -> Add2/2
  Shift Arithmetic/1 -> Add2/3
  [Vref1] -> Compare To Zero/1
  Add2/1 -> OriginalSector/1  "OriginalSector"
  Compare To Zero/1 -> Add2/1
  Compare To Zero1/1 -> Shift Arithmetic1/1
  Compare To Zero2/1 -> Shift Arithmetic/1

== system MCU_FOC/FOC/FOC/Subsystem/Normal/SVPWM/Subsystem/SVPWMCal/SectorTransfer ==
  note: 3 1 5 4 6 2
      | 1 2 3 4 5 6
  OriginalSector : Inport
  Constant : Constant  Value=[2 6 1 4 3 5]  OutDataTypeStr=uint8
  Selector : Selector  IndexOptions=Index vector (port)  Indices=[1 3]  OutputSizes=1
  realSector : Outport
  wires:
  OriginalSector/1 -> Selector/2
  Constant/1 -> Selector/1
  Selector/1 -> realSector/1  "realSector"

== system MCU_FOC/FOC/FOC/Subsystem/Normal/SVPWM/Subsystem/SVPWMCal/Subsystem ==
  T1 : Inport
  T2 : Inport  Port=2
  Compare To Zero : simulink/Logic and Bit Operations/Compare To Zero  relop=<  OutDataTypeStr=boolean
  Compare To Zero1 : simulink/Logic and Bit Operations/Compare To Zero  relop=<  OutDataTypeStr=boolean
  Constant : Constant  Value=0.0001  OutDataTypeStr=single
  OverModulation : Subsystem  Description=过调制
  Switch : Switch  Criteria=u2 ~= 0  SaturateOnIntegerOverflow=off  InputSameDT=off
  Switch1 : Switch  Criteria=u2 ~= 0  SaturateOnIntegerOverflow=off  InputSameDT=off
  T1Final : Outport
  T2Final : Outport  Port=2
  wires:
  T1/1 -> Switch/3, Compare To Zero/1
  Compare To Zero/1 -> Switch/2
  Constant/1 -> Switch1/1, Switch/1
  Compare To Zero1/1 -> Switch1/2
  T2/1 -> Switch1/3, Compare To Zero1/1
  Switch/1 -> OverModulation/1(T1_In)
  Switch1/1 -> OverModulation/2(T2_In)
  OverModulation/1(T1) -> T1Final/1
  OverModulation/2(T2) -> T2Final/1

== system MCU_FOC/FOC/FOC/Subsystem/Normal/SVPWM/Subsystem/SVPWMCal/SwitchTime ==
  T1Final : Inport
  T2Final : Inport  Port=2
  realSector : Inport  Port=3
  Add : Sum
  Add1 : Sum
  Constant : Constant  OutDataTypeStr=single
  Minus : Sum  Inputs=+--
  Shift Arithmetic : ArithShift  BitShiftNumber=2  BitShiftDirection=Right
  Shift Arithmetic1 : ArithShift  BitShiftNumber=1  BitShiftDirection=Right
  Shift Arithmetic2 : ArithShift  BitShiftNumber=1  BitShiftDirection=Right
  SwitchTimeCal : MATLAB Function  TreatAsAtomicUnit=on
  Tcm1 : Outport
  Tcm2 : Outport  Port=2
  Tcm3 : Outport  Port=3
  wires:
  T1Final/1 -> Shift Arithmetic1/1, Minus/2
  Constant/1 -> Minus/1
  Minus/1 -> Shift Arithmetic/1
  Shift Arithmetic/1 -> Add/1, [Ta]
  Shift Arithmetic1/1 -> Add/2
  Shift Arithmetic2/1 -> Add1/2
  Add/1 -> [Tb], Add1/1
  T2Final/1 -> Shift Arithmetic2/1, Minus/3
  Add1/1 -> [Tc]
  realSector/1 -> SwitchTimeCal/1(realSelector)
  [Ta] -> SwitchTimeCal/2(Ta)  "Ta"
  [Tb] -> SwitchTimeCal/3(Tb)  "Tb"
  [Tc] -> SwitchTimeCal/4(Tc)  "Tc"
  SwitchTimeCal/1(Tcm1) -> Tcm1/1  "Tcm1"
  SwitchTimeCal/2(Tcm2) -> Tcm2/1  "Tcm2"
  SwitchTimeCal/3(Tcm3) -> Tcm3/1  "Tcm3"

== system MCU_FOC/FOC/FOC/Subsystem/Normal/SVPWM/Subsystem/SVPWMCal/Subsystem/OverModulation ==
  T1_In : Inport
  T2_In : Inport  Port=2
  Add : Sum
  Compare To Constant : simulink/Logic and Bit Operations/Compare To Constant  relop=>  const=1  OutDataTypeStr=boolean
  Switch : Switch  Criteria=u2 ~= 0  SaturateOnIntegerOverflow=off  InputSameDT=off
  Switch1 : Switch  Criteria=u2 ~= 0  SaturateOnIntegerOverflow=off  InputSameDT=off
  T12 : Subsystem
  T1 : Outport
  T2 : Outport  Port=2
  wires:
  T1_In/1 -> Add/1, Switch/3, T12/1(T1_In)
  T2_In/1 -> T12/2(T2_In), Switch1/3, Add/2
  Add/1 -> Compare To Constant/1
  Compare To Constant/1 -> Switch/2, Switch1/2, T12/Enable
  Switch/1 -> T1/1
  Switch1/1 -> T2/1
  T12/1(T1) -> Switch/1
  T12/2(T2) -> Switch1/1

== system MCU_FOC/FOC/FOC/Subsystem/Normal/SVPWM/Subsystem/SVPWMCal/Subsystem/OverModulation/T12 ==
  T1_In : Inport
  T2_In : Inport  Port=2
  Enable : EnablePort
  MATLAB Function : MATLAB Function  TreatAsAtomicUnit=on
  T1 : Outport
  T2 : Outport  Port=2
  wires:
  T1_In/1 -> MATLAB Function/1(T1_In)
  T2_In/1 -> MATLAB Function/2(T2_In)
  MATLAB Function/1(T1) -> T1/1
  MATLAB Function/2(T2) -> T2/1

== stateflow chart MCU_FOC/FOC/Speed/Chart ==
  (default) -> (junction 1)
  (junction 1) -> (junction 16) : [PWMStep==4]
  (junction 16) -> (junction 18) : {index=0;}
  (junction 18) -> (junction 17) [order 1] : [index<40]
  (junction 17) -> (junction 19) : {PosDeltFilterArray[index] = PwmPrdchgCoffe*PosDeltFilterArray[index]}
  (junction 20) -> (junction 18)
  (junction 18) -> (junction 21) [order 2] : {
      | PosDeltFilterArray[PosDeltArrayCnt] = PosDelt;
      | PosDeltArrayCnt = PosDeltArrayCnt+1;
      | }
  (junction 19) -> (junction 20) : {index=index+1;}
  (junction 21) -> (junction 26) [order 2]
  (junction 21) -> (junction 26) [order 1] : [PosDeltArrayCnt>=40]{PosDeltArrayCnt=0}
  (junction 26) -> (junction 30)
  data: PosDeltFilterArray output int16 size=40; PWMStep input uint8; index local uint8 =0; PwmPrdchgCoffe input single; PosDelt input int16; PosDeltArrayCnt output uint16 =0

== matlab function MCU_FOC/FOC/FOC/Subsystem/Normal/SVPWM/Subsystem/SVPWMCal/SwitchTime/SwitchTimeCal ==
  data: realSelector input; Ta input; Tcm1 output; Tb input; Tc input; Tcm2 output; Tcm3 output
function [Tcm1,Tcm2,Tcm3] = TcmCal(realSelector,Ta,Tb,Tc)

tcm1 = single(0);
tcm2 = single(0);
tcm3 = single(0);

if realSelector == 1
    tcm1 = Ta;
    tcm2 = Tb;
    tcm3 = Tc;
elseif realSelector == 2
    tcm1 = Tb;
    tcm2 = Ta;
    tcm3 = Tc;
elseif realSelector == 3
    tcm1 = Tc;
    tcm2 = Ta;
    tcm3 = Tb;
elseif realSelector == 4
    tcm1 = Tc;
    tcm2 = Tb;
    tcm3 = Ta;
elseif realSelector == 5
    tcm1 = Tb;
    tcm2 = Tc;
    tcm3 = Ta;
elseif realSelector == 6
    tcm1 = Ta;
    tcm2 = Tc;
    tcm3 = Tb;

end
Tcm1 = tcm1;
Tcm2 = tcm2;
Tcm3 = tcm3;
end

== matlab function MCU_FOC/FOC/FOC/Subsystem/Normal/SVPWM/Subsystem/SVPWMCal/ActionTimeCal/ActionTimeJudgement ==
  data: realSector input; Ts input; X input; T1 output; Y input; Z input; T2 output
function [T1,T2] = judgement(realSector, Ts, X, Y, Z)

t1 = single(0);
t2 = single(0);
t0 = single(0);
t7 = single(0);

if realSector == 1

    t1 = -Z;
    t2 = X;


elseif realSector == 2

    t1 = Z;
    t2 = Y;


elseif realSector == 3
    t1 = X;
    t2 = -Y;


elseif realSector == 4

    t1 = -X;
    t2 = Z;


elseif realSector == 5

    t1 = -Y;
    t2 = -Z;


elseif realSector == 6

    t1 = Y;
    t2 = -X;

end


T1 = t1;
T2 = t2;
t0 = (Ts-t1-t2)/2;
t7 = (Ts-t1-t2)/2;

end

== stateflow chart MCU_FOC/FOC/FOC/Subsystem/Normal/IdqGiveCal/AgeingMode/Chart ==
  state Act = Slope(Ref,step) [function]
  (default) -> (junction 1)
  (junction 1) -> (junction 4) [order 1] : [Cnt < 10000]
  (junction 1) -> (junction 15) [order 2] : {
      | AgentFreq =Slope(WorkCmdTaskFreqCmd,0.00002);
      | Id = WorkCmdCoreIdCmd;
      | Iq = WorkCmdCoreIqCmd;
      | }
  (junction 4) -> (junction 6) : {
      | Cnt = Cnt +1;
      | Id = WorkCmdCoreCurrentCmd
      | Iq = 0;
      | }
  (junction 6) -> (junction 15)
  (junction 15) -> (junction 18)
  data: Ref function_input double size=1; step function_input double size=1; Act function_output; Cnt local uint16 size=1 =0; WorkCmdCoreCurrentCmd input; WorkCmdTaskFreqCmd input; Id output single =0; Iq output single; WorkCmdCoreIdCmd input; WorkCmdCoreIqCmd input; AgentFreq output single =0

== matlab function MCU_FOC/FOC/FOC/Subsystem/Normal/SVPWM/Subsystem/SVPWMCal/Subsystem/OverModulation/T12/MATLAB Function ==
  data: T1_In input single; T1 output single; T2_In input single; T2 output single
function [T1,T2] = fcn(T1_In, T2_In)

 if T1_In>1 && T1_In>T2_In
     T1 = single(1);
     T2 = single(0);

 elseif T2_In>1 && T2_In>T1_In
     T1 = single(0);
     T2 = single(1);
 else
     T1 = T1_In/(T1_In+T2_In);
     T2 = 1-T1;


end

== matlab function MCU_FOC/FOC/FOC/Subsystem/Normal/SVPWM/Subsystem/SVPWMCal/N Caculate/MATLAB Function ==
  data: u input; y output
function y = fcn(u)
if u==0
    y=1;
else
    y = u;
end

== matlab function MCU_FOC/FOC/FOC/Subsystem/Normal/SVPWM/Subsystem/DPWM/MATLAB Function ==
  data: TMin input; Ualpha input; Ta output; Ubeta input; Tb output; Tc output
function [Ta, Tb, Tc] = Sdpwm2_Gener_Calc(TMin, Ualpha, Ubeta)
% SVPWM计算函数（不连续调制模式），适用于Simulink MATLAB Function模块
% 输入强制转换为single类型，所有内部运算使用single精度
% 输入：
%   Ualpha : α轴电压标幺值（归一化到0~1之间）
%   Ubeta  : β轴电压标幺值
%   TMin   : 最小时间阈值（用于负时间钳位，通常设为0或小正数）
% 输出：
%   Ta, Tb, Tc : 三相占空比（范围0~1，single类型）

    % 将所有输入参数强制转换为single类型
    TMin   = single(TMin);
    Ualpha = single(Ualpha);
    Ubeta  = single(Ubeta);

    % 常数 sqrt(3)/2 定义为single
    SQRT3BY2 = single(0.8660254037844386);

    % 对TMin进行限幅（使用single常数）
    tmin_lim = TMin;
    if tmin_lim < single(0)
        tmin_lim = single(0);
    elseif tmin_lim > single(0.05)
        tmin_lim = single(0.05);
    end

    % 第一次计算 Va, Vb, Vc 用于扇区判断
    Va = Ubeta;
    Vb = -single(0.5) * Ubeta + SQRT3BY2 * Ualpha;
    Vc = -single(0.5) * Ubeta - SQRT3BY2 * Ualpha;

    % 扇区判定（按二进制加权）
    Sector = uint8(0);  % 使用整数类型，避免类型转换问题
    if Va > single(0)
        Sector = uint8(1);
    end
    if Vb > single(0)
        Sector = Sector + uint8(2);
    end
    if Vc > single(0)
        Sector = Sector + uint8(4);
    end

    % 第二次计算 X, Y, Z（仍用 Va, Vb, Vc 变量）
    Va = Ubeta;                          % X
    Vb = single(0.5) * Ubeta + SQRT3BY2 * Ualpha; % Y
    Vc = single(0.5) * Ubeta - SQRT3BY2 * Ualpha; % Z

    % 根据扇区计算 t1, t2 以及最终占空比
    switch Sector
        case 0  % 零矢量
            Ta = single(0.5);
            Tb = single(0.5);
            Tc = single(0.5);

        case 1  % 扇区1：t1=Z, t2=Y  (B相全通)
            t1 = Vc;
            t2 = Vb;
            [t1, t2] = clampAndScale(t1, t2, tmin_lim);
            Tb = single(0);
            Ta = Tb + t1;
            Tc = Ta + t2;

        case 2  % 扇区2：t1=Y, t2=-X (A相全通)
            t1 = Vb;
            t2 = -Va;
            [t1, t2] = clampAndScale(t1, t2, tmin_lim);
            Ta = single(0);
            Tc = Ta + t1;
            Tb = Tc + t2;

        case 3  % 扇区3：t1=-Z, t2=X  (C相全关)
            t1 = -Vc;
            t2 = Va;
            [t1, t2] = clampAndScale(t1, t2, tmin_lim);
            Ta = single(1) - t1 - t2;
            Tb = Ta + t1;
            Tc = single(1);

        case 4  % 扇区4：t1=-X, t2=Z  (C相全通)
            t1 = -Va;
            t2 = Vc;
            [t1, t2] = clampAndScale(t1, t2, tmin_lim);
            Tc = single(0);
            Tb = Tc + t1;
            Ta = Tb + t2;

        case 5  % 扇区5：t1=X, t2=-Y  (A相全关)
            t1 = Va;
            t2 = -Vb;
            [t1, t2] = clampAndScale(t1, t2, tmin_lim);
            Tb = single(1) - t1 - t2;
            Tc = Tb + t1;
            Ta = single(1);

        case 6  % 扇区6：t1=-Y, t2=-Z  (B相全关)
            t1 = -Vb;
            t2 = -Vc;
            [t1, t2] = clampAndScale(t1, t2, tmin_lim);
            Tc = single(1) - t1 - t2;
            Ta = Tc + t1;
            Tb = single(1);

        otherwise
            % 安全性处理，实际不会执行
            Ta = single(0.5);
            Tb = single(0.5);
            Tc = single(0.5);
    end
end

% -------------------------------------------------------------------------
function [t1, t2] = clampAndScale(t1, t2, TMin)
% 负时间钳位及过调制处理，所有输入和输出均为single类型

    % 负时间钳位（用TMin代替负值）
    if t1 < single(0)
        t1 = TMin;
    end
    if t2 < single(0)
        t2 = TMin;
    end

    % 过调制处理（t1+t2 > 1 时按比例缩放）
    if (t1 + t2) > single(1)
        if (t1 > single(1)) && (t1 > t2)
            t1 = single(1);
            t2 = single(0);
        elseif (t2 > single(1)) && (t2 > t1)
            t1 = single(0);
            t2 = single(1);
        else
            t1 = t1 / (t1 + t2);
            t2 = single(1) - t1;
        end
    end
end
